simulink model "example_simulink_LaserRangeFinder"  (Simulink 7.0)
settings: Solver=FixedStepDiscrete  StartTime=0.0  StopTime=inf  FixedStep=10  RelTol=1e-3
libraries: lib_robotinohardware x10, simulink x1
settings Model: Creator=indorewala  LastModifiedBy=ciesla

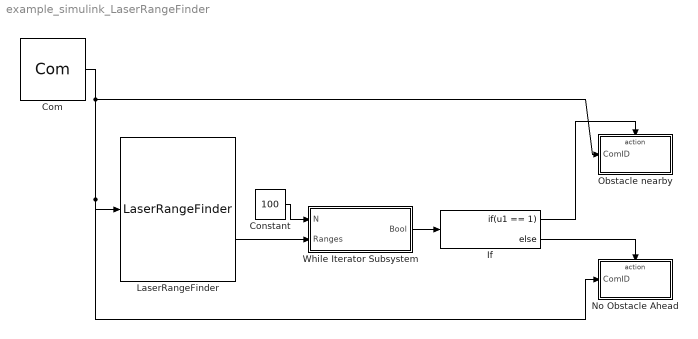
== system example_simulink_LaserRangeFinder ==
  Com : lib_robotinohardware/Com  ip='127.0.0.1'
  Constant : Constant  Value=100  OutDataType=sfix(16)  OutScaling=2^0
  If : If  IfExpression=u1 == 1
  LaserRangeFinder : lib_robotinohardware/LaserRangeFinder
  No Obstacle Ahead : Subsystem  TreatAsAtomicUnit=on
  Obstacle nearby : Subsystem  TreatAsAtomicUnit=on
  While Iterator Subsystem : Subsystem  TreatAsAtomicUnit=on
  wires:
  Com/1 -> Obstacle nearby/1(ComID), LaserRangeFinder/1, No Obstacle Ahead/1(ComID)
  If/2 -> No Obstacle Ahead/Action
  If/1 -> Obstacle nearby/Action
  While Iterator Subsystem/1(Bool) -> If/1
  LaserRangeFinder/10 -> While Iterator Subsystem/2(Ranges)
  Constant/1 -> While Iterator Subsystem/1(N)

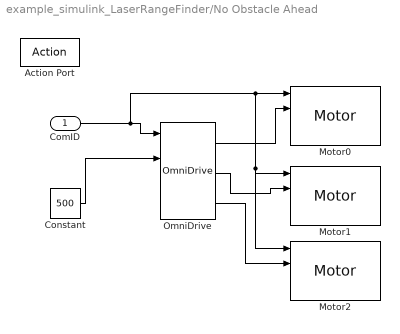
== system example_simulink_LaserRangeFinder/No Obstacle Ahead ==
  ComID : Inport  OutDataType=sfix(16)  OutScaling=2^0
  Action Port : ActionPort  ActionType=else
  Constant : Constant  Value=500  OutDataType=sfix(16)  OutScaling=2^0
  Motor0 : lib_robotinohardware/Motor  num=0  kp=0.9  ki=0.1  kd=0
  Motor1 : lib_robotinohardware/Motor  num=1  kp=0.9  ki=0.1  kd=0
  Motor2 : lib_robotinohardware/Motor  num=2  kp=0.9  ki=0.1  kd=0
  OmniDrive : lib_robotinohardware/OmniDrive
  wires:
  ComID/1 -> OmniDrive/1, Motor0/1, Motor2/1, Motor1/1
  Constant/1 -> OmniDrive/2
  OmniDrive/1 -> Motor0/2
  OmniDrive/2 -> Motor1/2
  OmniDrive/3 -> Motor2/2

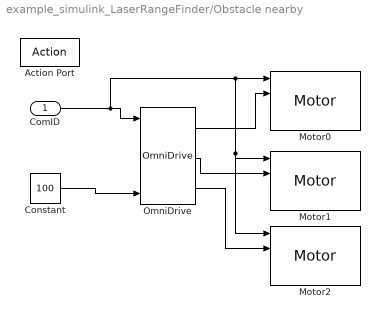
== system example_simulink_LaserRangeFinder/Obstacle nearby ==
  ComID : Inport  OutDataType=sfix(16)  OutScaling=2^0
  Action Port : ActionPort  ActionType=then
  Constant : Constant  Value=100  OutDataType=sfix(16)  OutScaling=2^0
  Motor0 : lib_robotinohardware/Motor  num=0  kp=0.9  ki=0.1  kd=0
  Motor1 : lib_robotinohardware/Motor  num=1  kp=0.9  ki=0.1  kd=0
  Motor2 : lib_robotinohardware/Motor  num=2  kp=0.9  ki=0.1  kd=0
  OmniDrive : lib_robotinohardware/OmniDrive
  wires:
  ComID/1 -> OmniDrive/1, Motor0/1, Motor1/1, Motor2/1
  Constant/1 -> OmniDrive/4
  OmniDrive/1 -> Motor0/2
  OmniDrive/2 -> Motor1/2
  OmniDrive/3 -> Motor2/2

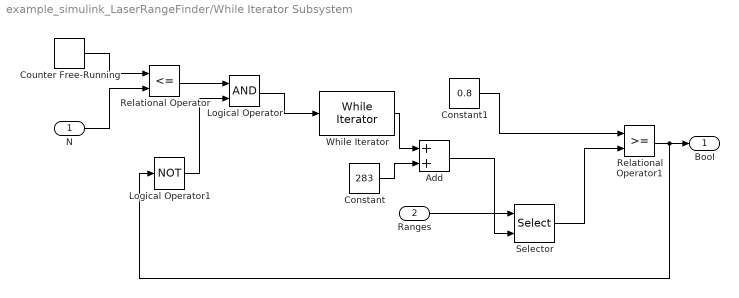
== system example_simulink_LaserRangeFinder/While Iterator Subsystem ==
  N : Inport  OutDataType=sfix(16)  OutScaling=2^0
  Ranges : Inport  Port=2  OutDataType=sfix(16)  OutScaling=2^0
  Add : Sum  OutDataType=sfix(16)  OutScaling=2^-10
  Constant : Constant  Value=283  OutDataType=sfix(16)  OutScaling=2^0
  Constant1 : Constant  Value=0.8  OutDataType=sfix(16)  OutScaling=2^0
  Counter Free-Running : simulink/Sources/Counter Free-Running  SystemSampleTime=-1  NumBits=16  tsamp=-1
  Logical Operator : Logic  AllPortsSameDT=off  OutDataTypeMode=boolean
  Logical Operator1 : Logic  Operator=NOT  AllPortsSameDT=off  OutDataTypeMode=boolean
  Relational Operator : RelationalOperator  Operator=<=  LogicOutDataTypeMode=boolean
  Relational Operator1 : RelationalOperator  LogicOutDataTypeMode=boolean
  Selector : Selector  InputPortWidth=1000  IndexOptions=Starting index (port)  Indices=[1 3]  OutputSizes=1
  While Iterator : WhileIterator  WhileBlockType=do-while  ShowIterationPort=on
  Bool : Outport  OutDataType=sfix(16)  OutScaling=2^0
  wires:
  Counter Free-Running/1 -> Relational Operator/1
  N/1 -> Relational Operator/2
  Relational Operator/1 -> Logical Operator/1
  Logical Operator/1 -> While Iterator/1
  Logical Operator1/1 -> Logical Operator/2
  While Iterator/1 -> Add/1
  Constant/1 -> Add/2
  Relational Operator1/1 -> Bool/1, Logical Operator1/1
  Constant1/1 -> Relational Operator1/1
  Ranges/1 -> Selector/1
  Add/1 -> Selector/2
  Selector/1 -> Relational Operator1/2
